simulink model "PV_array"  (R2022a)
settings: Solver=VariableStepAuto  StartTime=0.0  StopTime=10.0  RelTol=1e-3
libraries: spsControlledVoltageSourceLib x1, spsPVArrayLib x1, simulink x1, spspowerguiLib x1
settings Model: Creator=Home computer  LastModifiedBy=Home computer

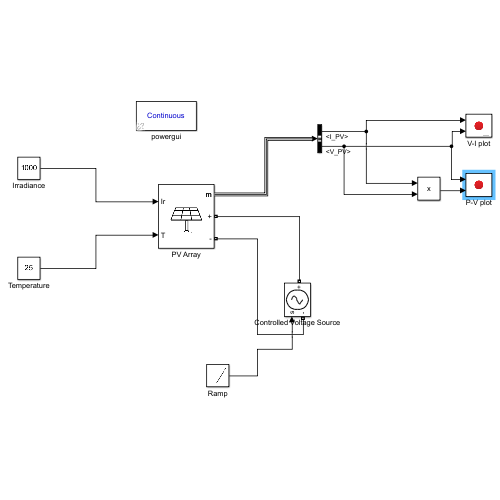
[thumbnail: Simulink's stored preview of the top-level diagram]
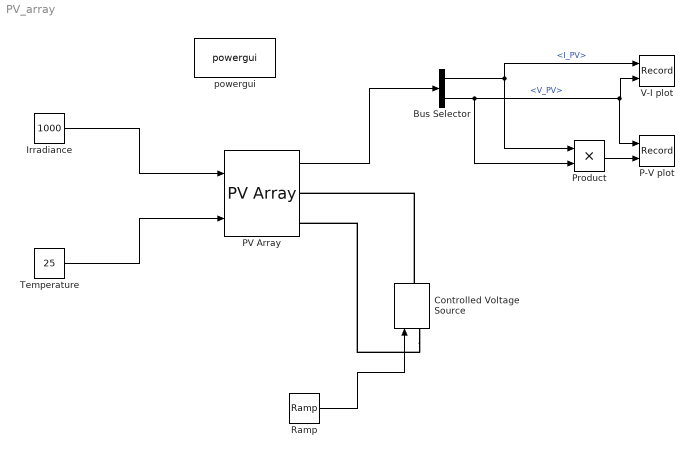
== system PV_array ==
  Bus Selector : BusSelector  OutputSignals=I_PV,V_PV
  Controlled Voltage Source : spsControlledVoltageSourceLib/Controlled Voltage Source  Initialize=on  Source_Type=AC  Amplitude=0  Phase=0  Frequency=0  Measurements=None
  Irradiance : Constant  Value=1000
  P-V plot : Record  FileSettingsInternal="{\"entries\":[{\"content\":{\"excelSettings\":{\"content\":{},\"type\":\"Streamout.ExcelSettings\"}},\"type\":\"Streamout.FileSettingStorage\",\"uuid\":\"e80199c9-27e7-4bb7-b21d-47fa4b59f221\"}],\"packageUris\":[\"http://schema.mathworks.com/mf0/streamout_blocks/R2020a\"],\"version\":\"1.0\"}"  Layout=[1 1]  SignalsInternal="{\"entries\":[{\"content\":{\"signals\":[{\"content\":{\"blockPath\":[\"untitled/P-V plot\"],\"channel\":[],\"dimensions\":[1],\"domain\":\"untitled/P-V plot\",\"lineColor\":\"#77ac30\",\"plots\":[],\"port\":1,\"sid\":[\"\"],\"signalID\":355,\"signalName\":\"<V_PV>\"},\"type\":\"RecordBlkView.Signal\",\"uuid\":\"ed5ac6eb-6039-42ab-b436-47866664b7f3\"},{\"content\":{\"blockPath\":[\"untitled/P-V plot\"],\"channel\":[],\"dimensions\":[1],\"domain\":\"untitled/P-V plot\",\"lineColor\":\"#4dbeee\",\"plots\":[],\"port\":2,\"sid\":[\"\"],\"signalID\":359,\"signalName\":\"Product\"},\"type\":\"RecordBlkView.Signal\",\"uuid\":\"e819d7c1-bd02-44d7-87e9-e239fa642a54\"}]},\"type\":\"RecordBlkView.InputSignals\",\"uuid\":\"e2401d25-8a91-4699-a1b4-388a2d05a65f\"}],\"packageUris\":[\"http://schema.mathworks.com/mf0/streamout_blocks/R2020a\"],\"version\":\"1.0\"}"  VisualizationBindings="{\"xyplotplugin\":{\"info\":[{\"series\":[],\"subplotID\":1}]}}"  CompatibilityTag=XY
  PV Array : spsPVArrayLib/PV Array  Npar=1  Nser=1  PlotType=array @ 1000 W/m2 & specified temperatures  S_vec="[ 1000  500  100 ]"  Temp_C_vec="[ 45 25  ]"  ModuleName=SunPower SER-220P  PlotWhenSelected=off  Pm=219.9716  Ncell=60  Voc=36.3  Isc=8.3  Vm=29.02  Im=7.58  beta_Voc_pc=-0.355  alpha_Isc_pc=0.043795  beta_Voc=-0.12887  alpha_Isc=0.003635  IL=8.3331  I0=2.2776e-10  nI=0.97001  Rsh=95.1238  Rs=0.37924  RobustModel=off  RobustCellTemperature=313.3991  BAL=on  Tc=1e-6  Tfilter=5e-5
  Product : Product
  Ramp : simulink/Sources/Ramp  slope=1  start=0  InitialOutput=0
  Temperature : Constant  Value=25
  V-I plot : Record  FileSettingsInternal="{\"entries\":[{\"content\":{\"excelSettings\":{\"content\":{},\"type\":\"Streamout.ExcelSettings\"}},\"type\":\"Streamout.FileSettingStorage\",\"uuid\":\"8f6d3354-2ac3-4b83-a8f9-ebf19e72b692\"}],\"packageUris\":[\"http://schema.mathworks.com/mf0/streamout_blocks/R2020a\"],\"version\":\"1.0\"}"  Layout=[1 1]  SignalsInternal="{\"entries\":[{\"content\":{\"signals\":[{\"content\":{\"blockPath\":[\"untitled/V-I plot\"],\"channel\":[],\"dimensions\":[1],\"domain\":\"untitled/V-I plot\",\"lineColor\":\"#a2142f\",\"plots\":[],\"port\":1,\"sid\":[\"\"],\"signalID\":363,\"signalName\":\"<I_PV>\"},\"type\":\"RecordBlkView.Signal\",\"uuid\":\"830d08e5-8c6c-4360-bbe4-f26f469f9ad3\"},{\"content\":{\"blockPath\":[\"untitled/V-I plot\"],\"channel\":[],\"dimensions\":[1],\"domain\":\"untitled/V-I plot\",\"lineColor\":\"#139fff\",\"plots\":[],\"port\":2,\"sid\":[\"\"],\"signalID\":367,\"signalName\":\"<V_PV>\"},\"type\":\"RecordBlkView.Signal\",\"uuid\":\"97a38ed0-f8ee-4fc0-b495-8ec52dd64092\"}]},\"type\":\"RecordBlkView.InputSignals\",\"uuid\":\"dbdbf925-6dc1-4e29-9222-4fa147bf80aa\"}],\"packageUris\":[\"http://schema.mathworks.com/mf0/streamout_blocks/R2020a\"],\"version\":\"1.0\"}"  VisualizationBindings="{\"xyplotplugin\":{\"info\":[{\"series\":[],\"subplotID\":1}]}}"  CompatibilityTag=XY
  powergui : spspowerguiLib/powergui  Priority=1  SimulationMode=Continuous  SampleTime=50e-6  frequency=60  Iterations=50  frequencyindice=0  Pbase=100e6  ErrMax=1e-4  UnitsV=kV  UnitsW=MW  buscounter=0  FunctionMessages=off  echomessages=off  EnableUseOfTLC=off  CurrentSourceSwitches=off  DisableSnubberDevices=off  DisableRonSwitches=off  DisableVfSwitches=off  DisplayEquations=off  AutomaticDiscreteSolvers=off  SolverType=Tustin/Backward Euler (TBE)  Interpol=off  ExternalGateDelay=off  methode=off  Ts=100  x0status=blocks  SPID=on  SwTol=0  HookPort=off  NonlinearTolerance=1e-4  nMaxIteration=100  ContinueOnMaxIteration=off  RestoreLinks=warning  ResistiveCurrentMeasurement=off  Frange=[0:2:500]  Ylog=off  Xlog=on  ShowGrid=off  save=off  variable=ZData  structure=0  ZoomFFT=off  StartTime=0.0  cycles=1  DisplayStyle=1  fundamental=60  FreqAxis=off  MaxFrequency=1000  frequencyindicesteady=1  RmsSteady=1  display=off
  wires:
  Irradiance/1 -> PV Array/1
  Temperature/1 -> PV Array/2
  Ramp/1 -> Controlled Voltage Source/1
  Bus Selector/1 -> Product/1, V-I plot/1  "<I_PV>"
  Bus Selector/2 -> P-V plot/1, V-I plot/2, Product/2  "<V_PV>"
  Product/1 -> P-V plot/2
  PV Array/1 -> Bus Selector/1
  connections:
  Controlled Voltage Source/LConn1 -- PV Array/RConn2
  Controlled Voltage Source/RConn1 -- PV Array/RConn1
